simulink model "mcb_hall_offset_host"  (R2021a)
settings: Solver=FixedStepDiscrete  StartTime=0.0  StopTime=inf  RelTol=1e-3  EnableMultiTasking=on
StartFcn:
  | set_param([bdroot '/Serial Communication/Emergency Stop'], 'Value', '1');
values from neighbouring files (symbols this model uses):
  Ts_uart = 0.01    [mcb_pmsm_foc_hall_MCSPTE1AK144_data.m]
undefined symbols (not defined in the file or in its folder): pmsm
libraries: simulink x6, mcbhostblockslib x3, mcbcontrolslib x2, mcbpositiondecoderlib x1
settings Model: Creator=The MathWorks, Inc.  LastModifiedBy=Prasad Hegde
settings SolverCC: AlgebraicLoopSolver=TrustRegion
settings DataIOCC: LimitDataPoints=on  SaveFormat=Array  ReturnWorkspaceOutputs=off
settings OptimizationCC: LifeSpan=1  EfficientTunableParamExpr=on
settings DebuggingCC: MergeDetectMultiDrivingBlocksExec=none  SolverPrmCheckMsg=warning  ParameterPrecisionLossMsg=none  AllowSymbolicDim=off  PregeneratedLibrarySubsystemCodeDiagnostic=none  SFUnexpectedBacktrackingDiag=warning  SFNoUnconditionalDefaultTransitionDiag=warning  SFExecutionAtInitializationDiag=none  SFMachineParentedDataDiag=warning  ArithmeticOperatorsInVariantConditions=warning
settings HardwareCC: ProdBitPerPointer=32  ProdLargestAtomicFloat=None  ProdIntDivRoundTo=Undefined  ProdEndianess=Unspecified  ProdWordSize=32  ProdHWDeviceType=32-bit Generic
settings ModelReferenceCC: PropagateSignalLabelsOutOfModel=off
settings SFSimCC: SimUseLocalCustomCode=off  MATLABDynamicMemAlloc=off
settings RTWCC: Description=Real-Time Workshop Embedded Coder  SystemTargetFile=ert.tlc  TemplateMakefile=ert_default_tmf  GenerateReport=on  RTWUseLocalCustomCode=off  IncludeHyperlinkInReport=on  LaunchReport=on  GenerateTraceInfo=on  GenerateTraceReport=on  GenerateTraceReportSl=on  GenerateTraceReportSf=on  GenerateTraceReportEml=on
settings CodeAppCC: IgnoreCustomStorageClasses=off  StateflowObjectComments=on  InternalIdentifier=Classic
settings ERTTargetCC: MultiwordLength=2048  GenerateSampleERTMain=on  ERTCustomFileTemplate=example_file_process.tlc  ConvertIfToSwitch=off  SuppressUnreachableDefaultCases=off
settings ConfigComp: CovMetricSettings=dw  CovSaveCumulativeToWorkspaceVar=on  CovSaveSingleToWorkspaceVar=on  CovExternalEMLEnable=off  CovSFcnEnable=off

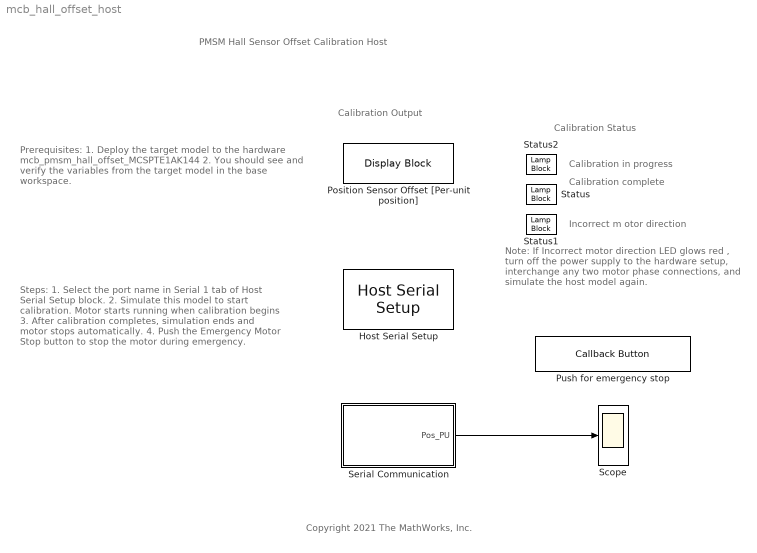
== system mcb_hall_offset_host ==
  note: PMSM Hall Sensor Offset Calibration Host
  note: Calibration Output
  note: Calibration Status
  note: Calibration in progress
  note: Calibration complete
  note: Incorrect m otor direction
  note: Steps:
      | 1. Select the port name in Serial 1 tab of
      | Host Serial Setup block.
      | 2. Simulate this model to start calibration.
      | Motor starts running when calibration
      | begins
      | 3. After calibration completes, simulation
      | ends and motor stops automatically.
      | 4. Push the Emergency Motor Stop button
      | to stop the motor during emergency.
  note: Prerequisites:
      | 1. Deploy the target model to the hardware
      | mcb_pmsm_hall_offset_MCSPTE1AK144
      |
      | 2. You should see and verify the variables
      | from the target model in the base
      | workspace.
  note: Note:
      | If Incorrect motor direction LED glows red , turn off the power supply to the hardware setup, interchange any two motor phase connections, and simulate the host model again.
  note: Copyright 2021 The MathWorks, Inc.
  Host Serial Setup : mcbhostblockslib/Host Serial Setup  Priority=-99  comPortSer1='Please_select_a_port'  baudRateA=256000  charLenA=8  stopBitA=1  parityA=none  timeoutA=2  ByteOrderA=LittleEndian  comPortSer2='Please_select_a_port'  baudRateB=115200  charLenB=8  stopBitB=1  parityB=none  timeoutB=1.0  ByteOrderB=LittleEndian  comPortSer3='Please_select_a_port'  baudRateC=115200  charLenC=8  stopBitC=1  parityC=none  timeoutC=1.0  ByteOrderC=LittleEndian  comPortSer4='Please_select_a_port'  baudRateD=115200  charLenD=8  stopBitD=1  parityD=none  timeoutD=1.0  ByteOrderD=LittleEndian
      settings: SourceProductBaseCode=MT
  Position Sensor Offset [Per-unit position] : DisplayBlock  LabelPosition=Hide  Format=short  Transparency=1
  Push for emergency stop : CallbackButton  ButtonText=Emergency Motor Stop
      settings: ClickFcn=set_param([bdroot '/Serial Communication/Emergency Stop'], 'Value', '0');
  Scope : Scope
  Serial Communication : Subsystem
  Status : LampBlock  LabelPosition=Hide
  Status1 : LampBlock  LabelPosition=Hide
  Status2 : LampBlock  LabelPosition=Hide
  wires:
  Serial Communication/1(Pos_PU) -> Scope/1

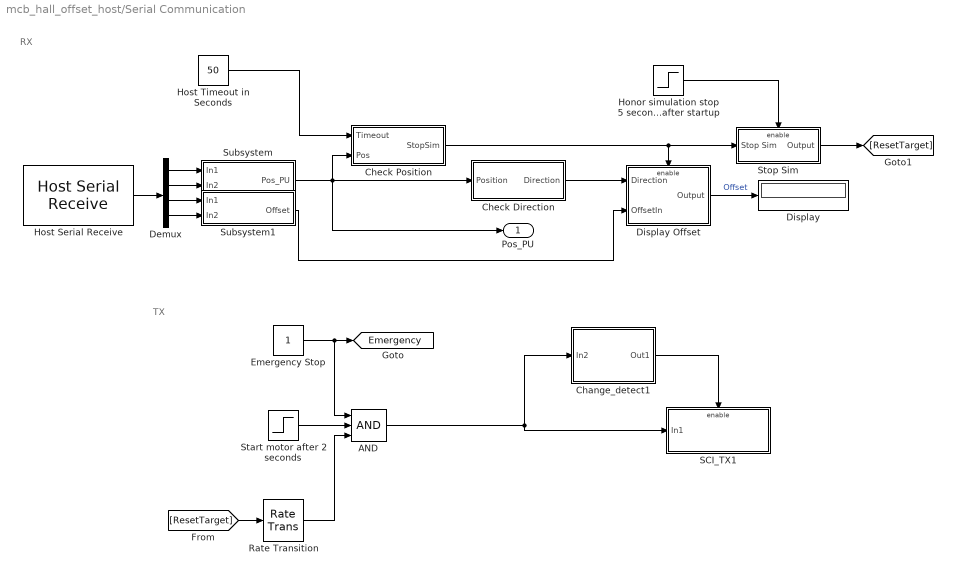
== system mcb_hall_offset_host/Serial Communication ==
  note: RX
  note: TX
  AND : Logic  Inputs=3  IconShape=distinctive  AllPortsSameDT=off  OutDataTypeStr=boolean
  Change_detect1 : Subsystem
  Check Direction : Subsystem
  Check Position : Subsystem
  Demux : Demux
  Display : Display
  Display Offset : Subsystem
  Emergency Stop : Constant  OutDataTypeStr=Inherit: Inherit via back propagation
  Honor simulation stop 5 seconds after startup : Step  Time=5  SampleTime=Ts_uart
  Host Serial Receive : mcbhostblockslib/Host Serial Receive  serialCon=Serial 1  dataHead='S'  dataTail='E'  dataType=uint8  dataDim=4  initValue=5  errOption=Output custom value  errValue=15  sampleTime=Ts_uart  outputStatus=off  blockingMode=on
      settings: SourceProductBaseCode=MT
  Host Timeout in Seconds : Constant  Value=50  OutDataTypeStr=Inherit: Inherit via back propagation
  Rate Transition : RateTransition
  SCI_TX1 : Subsystem  TreatAsAtomicUnit=on
  Start motor after 2 seconds : Step  Time=2  OutDataTypeStr=single  SampleTime=Ts_uart
  Stop Sim : Subsystem
  Subsystem : Subsystem
  Subsystem1 : Subsystem
  Pos_PU : Outport
  tag scope: Emergency=global
  wires:
  AND/1 -> Change_detect1/1(In2), SCI_TX1/1(In1)
  Host Serial Receive/1 -> Demux/1
  Change_detect1/1(Out1) -> SCI_TX1/Enable
  Emergency Stop/1 -> AND/1, [Emergency]
  Start motor after 2 seconds/1 -> AND/2
  Host Timeout in Seconds/1 -> Check Position/1(Timeout)
  Check Direction/1(Direction) -> Display Offset/1(Direction)
  Display Offset/1(Output) -> Display/1  "Offset"
  Demux/1 -> Subsystem/1(In1)
  Demux/2 -> Subsystem/2(In2)
  Demux/3 -> Subsystem1/1(In1)
  Demux/4 -> Subsystem1/2(In2)
  Subsystem/1(Pos_PU) -> Check Direction/1(Position), Pos_PU/1, Check Position/2(Pos)
  Honor simulation stop 5 seconds after startup/1 -> Stop Sim/Enable
  Rate Transition/1 -> AND/3
  Check Position/1(StopSim) -> Stop Sim/1(Stop Sim), Display Offset/Enable
  Subsystem1/1(Offset) -> Display Offset/2(OffsetIn)
  Stop Sim/1(Output) -> [ResetTarget]
  [ResetTarget] -> Rate Transition/1

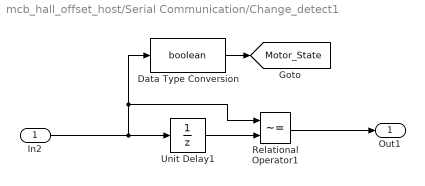
== system mcb_hall_offset_host/Serial Communication/Change_detect1 ==
  In2 : Inport
  Data Type Conversion : DataTypeConversion  OutDataTypeStr=boolean  RndMeth=Simplest
  Relational Operator1 : RelationalOperator  Operator=~=  OutDataTypeStr=boolean  RndMeth=Nearest
  Unit Delay1 : UnitDelay  SampleTime=-1  HasFrameUpgradeWarning=on
  Out1 : Outport  VectorParamsAs1DForOutWhenUnconnected=off
  tag scope: Motor_State=global
  wires:
  In2/1 -> Data Type Conversion/1, Relational Operator1/1, Unit Delay1/1
  Unit Delay1/1 -> Relational Operator1/2
  Relational Operator1/1 -> Out1/1
  Data Type Conversion/1 -> [Motor_State]

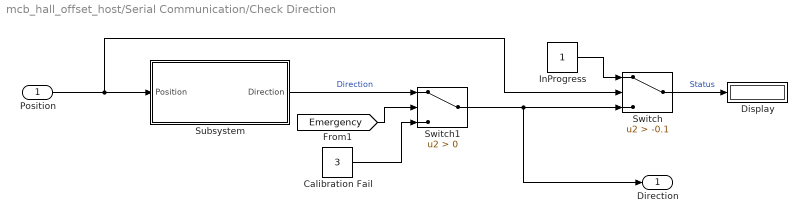
== system mcb_hall_offset_host/Serial Communication/Check Direction ==
  Position : Inport
  Calibration Fail : Constant  Value=3  OutDataTypeStr=uint16
  Display : Display
  InProgress : Constant  OutDataTypeStr=uint16
  Subsystem : Subsystem
  Switch : Switch  Criteria=u2 > Threshold  Threshold=-0.1
  Switch1 : Switch  Criteria=u2 > Threshold
  Direction : Outport
  wires:
  Subsystem/1(Direction) -> Switch1/1  "Direction"
  Switch1/1 -> Direction/1, Switch/3
  Calibration Fail/1 -> Switch1/3
  [Emergency] -> Switch1/2
  InProgress/1 -> Switch/1
  Position/1 -> Subsystem/1(Position), Switch/2
  Switch/1 -> Display/1  "Status"

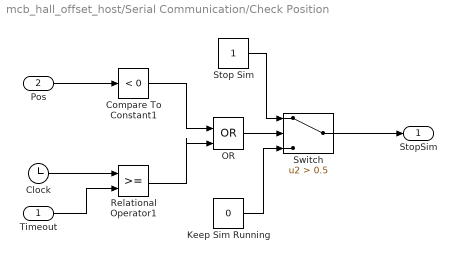
== system mcb_hall_offset_host/Serial Communication/Check Position ==
  Timeout : Inport
  Pos : Inport  Port=2
  Clock : Clock
  Compare To Constant1 : simulink/Logic and Bit Operations/Compare To Constant  relop=<  const=0  OutDataTypeStr=boolean
  Keep Sim Running : Constant  Value=0  OutDataTypeStr=Inherit: Inherit via back propagation
  OR : Logic  Operator=OR  IconShape=distinctive  AllPortsSameDT=off  OutDataTypeStr=boolean
  Relational Operator1 : RelationalOperator  OutDataTypeStr=boolean  RndMeth=Simplest
  Stop Sim : Constant  OutDataTypeStr=Inherit: Inherit via back propagation
  Switch : Switch  Criteria=u2 > Threshold  Threshold=0.5
  StopSim : Outport
  wires:
  Timeout/1 -> Relational Operator1/2
  Stop Sim/1 -> Switch/1
  Keep Sim Running/1 -> Switch/3
  OR/1 -> Switch/2
  Clock/1 -> Relational Operator1/1
  Relational Operator1/1 -> OR/2
  Compare To Constant1/1 -> OR/1
  Switch/1 -> StopSim/1
  Pos/1 -> Compare To Constant1/1

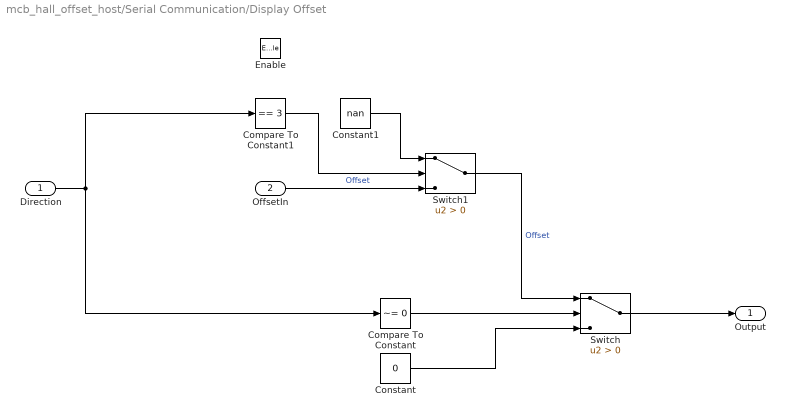
== system mcb_hall_offset_host/Serial Communication/Display Offset ==
  Direction : Inport
  OffsetIn : Inport  Port=2
  Enable : EnablePort
  Compare To Constant : simulink/Logic and Bit Operations/Compare To Constant  relop=~=  const=0  OutDataTypeStr=boolean
  Compare To Constant1 : simulink/Logic and Bit Operations/Compare To Constant  relop===  const=3  OutDataTypeStr=boolean
  Constant : Constant  Value=0  OutDataTypeStr=Inherit: Inherit via back propagation
  Constant1 : Constant  Value=nan  OutDataTypeStr=Inherit: Inherit via back propagation
  Switch : Switch  Criteria=u2 > Threshold
  Switch1 : Switch  Criteria=u2 > Threshold
  Output : Outport
  wires:
  Constant1/1 -> Switch1/1
  Compare To Constant1/1 -> Switch1/2
  Compare To Constant/1 -> Switch/2
  OffsetIn/1 -> Switch1/3  "Offset"
  Direction/1 -> Compare To Constant1/1, Compare To Constant/1
  Switch1/1 -> Switch/1  "Offset"
  Constant/1 -> Switch/3
  Switch/1 -> Output/1

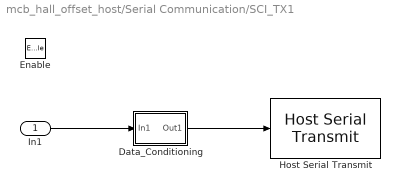
== system mcb_hall_offset_host/Serial Communication/SCI_TX1 ==
  In1 : Inport
  Enable : EnablePort
  Data_Conditioning : Subsystem
  Host Serial Transmit : mcbhostblockslib/Host Serial Transmit  serialCon=Serial 1  header=''  tail=''  enableBlockingMode=off
      settings: SourceProductBaseCode=MT
  wires:
  In1/1 -> Data_Conditioning/1(In1)
  Data_Conditioning/1(Out1) -> Host Serial Transmit/1

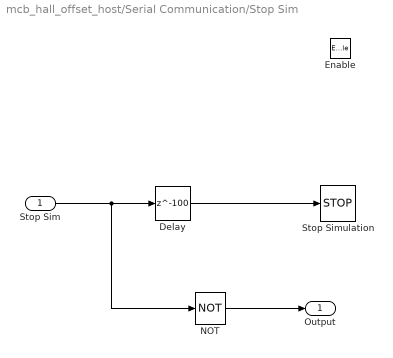
== system mcb_hall_offset_host/Serial Communication/Stop Sim ==
  Stop Sim : Inport
  Enable : EnablePort
  Delay : Delay  DelayLength=100
  NOT : Logic  Operator=NOT  IconShape=distinctive  AllPortsSameDT=off  OutDataTypeStr=boolean
  Stop Simulation : Stop
  Output : Outport  InitialOutput=1
  wires:
  Stop Sim/1 -> NOT/1, Delay/1
  Delay/1 -> Stop Simulation/1
  NOT/1 -> Output/1

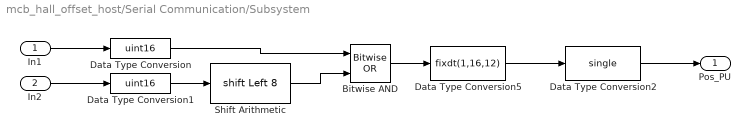
== system mcb_hall_offset_host/Serial Communication/Subsystem ==
  In1 : Inport
  In2 : Inport  Port=2
  Bitwise AND : simulink/Logic and Bit Operations/Bitwise Operator  logicop=OR  UseBitMask=off  NumInputPorts=2  BitMask=bin2dec('11011001')  BitMaskRealWorld=Stored Integer
  Data Type Conversion : DataTypeConversion  OutDataTypeStr=uint16  RndMeth=Simplest
  Data Type Conversion1 : DataTypeConversion  OutDataTypeStr=uint16  RndMeth=Simplest
  Data Type Conversion2 : DataTypeConversion  OutDataTypeStr=single  RndMeth=Simplest
  Data Type Conversion5 : DataTypeConversion  OutDataTypeStr=fixdt(1,16,12)  ConvertRealWorld=Stored Integer (SI)  RndMeth=Simplest
  Shift Arithmetic : ArithShift  BitShiftNumber=8  BitShiftDirection=Left
  Pos_PU : Outport
  wires:
  In1/1 -> Data Type Conversion/1
  Data Type Conversion5/1 -> Data Type Conversion2/1
  In2/1 -> Data Type Conversion1/1
  Shift Arithmetic/1 -> Bitwise AND/2
  Bitwise AND/1 -> Data Type Conversion5/1
  Data Type Conversion1/1 -> Shift Arithmetic/1
  Data Type Conversion/1 -> Bitwise AND/1
  Data Type Conversion2/1 -> Pos_PU/1

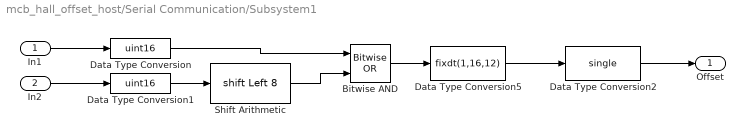
== system mcb_hall_offset_host/Serial Communication/Subsystem1 ==
  In1 : Inport
  In2 : Inport  Port=2
  Bitwise AND : simulink/Logic and Bit Operations/Bitwise Operator  logicop=OR  UseBitMask=off  NumInputPorts=2  BitMask=bin2dec('11011001')  BitMaskRealWorld=Stored Integer
  Data Type Conversion : DataTypeConversion  OutDataTypeStr=uint16  RndMeth=Simplest
  Data Type Conversion1 : DataTypeConversion  OutDataTypeStr=uint16  RndMeth=Simplest
  Data Type Conversion2 : DataTypeConversion  OutDataTypeStr=single  RndMeth=Simplest
  Data Type Conversion5 : DataTypeConversion  OutDataTypeStr=fixdt(1,16,12)  ConvertRealWorld=Stored Integer (SI)  RndMeth=Simplest
  Shift Arithmetic : ArithShift  BitShiftNumber=8  BitShiftDirection=Left
  Offset : Outport
  wires:
  Data Type Conversion/1 -> Bitwise AND/1
  Data Type Conversion1/1 -> Shift Arithmetic/1
  Bitwise AND/1 -> Data Type Conversion5/1
  Shift Arithmetic/1 -> Bitwise AND/2
  In2/1 -> Data Type Conversion1/1
  Data Type Conversion5/1 -> Data Type Conversion2/1
  In1/1 -> Data Type Conversion/1
  Data Type Conversion2/1 -> Offset/1

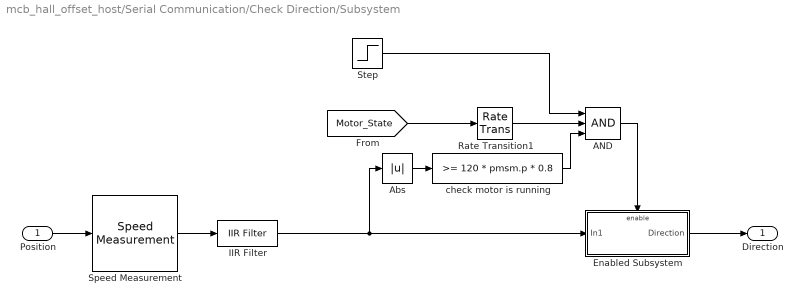
== system mcb_hall_offset_host/Serial Communication/Check Direction/Subsystem ==
  Position : Inport
  AND : Logic  Inputs=3  IconShape=distinctive  AllPortsSameDT=off  OutDataTypeStr=boolean
  Abs : Abs
  Enabled Subsystem : Subsystem  TreatAsAtomicUnit=on
  IIR Filter : mcbcontrolslib/IIR Filter  VariantControl=Low Pass Filter  VariantSelect=Low-pass  Filter_constant=0.01  advancedSettings=off  Ts=50e-6  cutOff_freq=32.1525
      settings: SourceProductBaseCode=MT
  Rate Transition1 : RateTransition
  Speed Measurement : mcbpositiondecoderlib/Speed Measurement  PositionUnit=Per unit  SpeedCalculationMode=Maximum application speed  SampleTimeAsync=Ts_uart  MaximumApplicationSpeed=4000  SpeedResolution=5e-6  DelayLength=1  MaximumMeasurableSpeed=1500  MeasurableSpeedResolution=6.9849e-07  SpeedUnit=RPM  PerUnitSpeed=1000  SpeedDataType=single
      settings: SourceProductBaseCode=MT
  Step : Step  Time=5  SampleTime=Ts_uart
  check motor is running : simulink/Logic and Bit Operations/Compare To Constant  relop=>=  const=120 * pmsm.p * 0.8  OutDataTypeStr=boolean
  Direction : Outport
  wires:
  Step/1 -> AND/1
  Position/1 -> Speed Measurement/1
  Rate Transition1/1 -> AND/2
  AND/1 -> Enabled Subsystem/Enable
  Enabled Subsystem/1(Direction) -> Direction/1
  Speed Measurement/1 -> IIR Filter/1
  [Motor_State] -> Rate Transition1/1
  Abs/1 -> check motor is running/1
  IIR Filter/1 -> Abs/1, Enabled Subsystem/1(In1)
  check motor is running/1 -> AND/3

== system mcb_hall_offset_host/Serial Communication/SCI_TX1/Data_Conditioning ==
  In1 : Inport
  Data Type Conversion : DataTypeConversion  OutDataTypeStr=uint8  RndMeth=Simplest
  Out1 : Outport  VectorParamsAs1DForOutWhenUnconnected=off
  wires:
  Data Type Conversion/1 -> Out1/1
  In1/1 -> Data Type Conversion/1

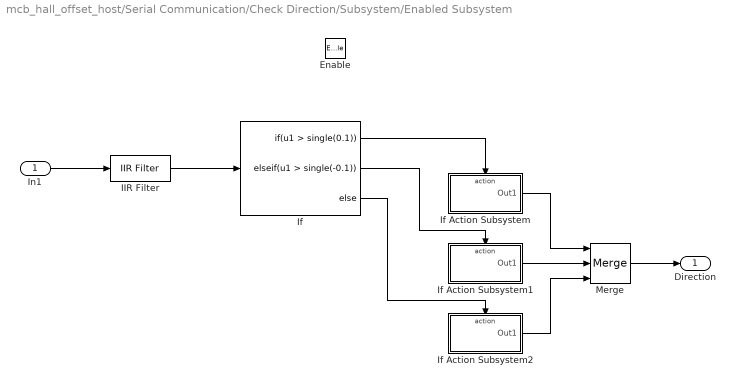
== system mcb_hall_offset_host/Serial Communication/Check Direction/Subsystem/Enabled Subsystem ==
  In1 : Inport
  Enable : EnablePort
  IIR Filter : mcbcontrolslib/IIR Filter  VariantControl=Low Pass Filter  VariantSelect=Low-pass  Filter_constant=0.001  advancedSettings=off  Ts=50e-6  cutOff_freq=3.1863
      settings: SourceProductBaseCode=MT
  If : If  IfExpression=u1 > single(0.1)  ElseIfExpressions=u1 > single(-0.1)
  If Action Subsystem : Subsystem  TreatAsAtomicUnit=on
  If Action Subsystem1 : Subsystem  TreatAsAtomicUnit=on
  If Action Subsystem2 : Subsystem  TreatAsAtomicUnit=on
  Merge : Merge  Inputs=3
  Direction : Outport
  wires:
  IIR Filter/1 -> If/1
  Merge/1 -> Direction/1
  If Action Subsystem2/1(Out1) -> Merge/3
  If Action Subsystem1/1(Out1) -> Merge/2
  If Action Subsystem/1(Out1) -> Merge/1
  If/3 -> If Action Subsystem2/Action
  If/2 -> If Action Subsystem1/Action
  If/1 -> If Action Subsystem/Action
  In1/1 -> IIR Filter/1

== system mcb_hall_offset_host/Serial Communication/Check Direction/Subsystem/Enabled Subsystem/If Action Subsystem ==
  Action Port : ActionPort  ActionPortLabel=if(u1 > single(0.1))
  Motor rotating in correct direction : Constant  Value=2  OutDataTypeStr=uint16
  Out1 : Outport
  wires:
  Motor rotating in correct direction/1 -> Out1/1

== system mcb_hall_offset_host/Serial Communication/Check Direction/Subsystem/Enabled Subsystem/If Action Subsystem1 ==
  Action Port : ActionPort  ActionPortLabel=elseif(u1 > single(-0.1))
  Motor not rotating : Constant  Value=0  OutDataTypeStr=uint16
  Out1 : Outport
  wires:
  Motor not rotating/1 -> Out1/1

== system mcb_hall_offset_host/Serial Communication/Check Direction/Subsystem/Enabled Subsystem/If Action Subsystem2 ==
  Action Port : ActionPort  ActionPortLabel=else
  Motor rotating in wrong direction : Constant  Value=3  OutDataTypeStr=uint16
  Out1 : Outport
  wires:
  Motor rotating in wrong direction/1 -> Out1/1
